simulink model "EV_compensated_system_via_detailed"  (R2016a)
settings: Solver=ode15s  StartTime=0.0  StopTime=tstop  MaxStep=1e-3  RelTol=1e-3
values from neighbouring files (symbols this model uses):
  Av = 2.16    [sim_parameters_via_motor_eff_data_improved.m]
  C = 500e-6    (= 0.0005)    [sim_parameters_via_motor_eff_data_improved.m]
  Cd = 0.26    [sim_parameters_via_motor_eff_data_improved.m]
  Cnom = 10    [sim_parameters_via_motor_eff_data_improved.m]
  Cr = 0.01    [sim_parameters_via_motor_eff_data_improved.m]
  etaC = 0.995    [sim_parameters_via_motor_eff_data_improved.m]
  Fv_max = Te_max*gratio/rw    (= 3970)    [sim_parameters_via_motor_eff_data_improved.m]
  Gci0 = Gciwc/abs(1+wzc/(i*wc))    [sim_parameters_via_motor_eff_data_improved.m]
  Gcm = 1000    [sim_parameters_via_motor_eff_data_improved.m]
  Gcv0 = Gcvwv/abs(1+wzo/(i*wv))    [sim_parameters_via_motor_eff_data_improved.m]
  gratio = 7.94    [sim_parameters_via_motor_eff_data_improved.m]
  H = 1/100    (= 0.01)    [sim_parameters_via_motor_eff_data_improved.m]
  Kp = Gciabs1/abs(1+wz1/(2*pi*10))    [sim_parameters_via_motor_eff_data_improved.m]
  L = 150e-6    (= 0.00015)    [sim_parameters_via_motor_eff_data_improved.m]
  L1 = 0.5e-3    (= 0.0005)    [sim_parameters_via_motor_eff_data_improved.m]
  lambda_m = 0.125    [sim_parameters_via_motor_eff_data_improved.m]
  Mp = 3    [sim_parameters_via_motor_eff_data_improved.m]
  Mv = 1250 + 55 + 15 + Ns*Mp*weight_cell    (= 1470)    [sim_parameters_via_motor_eff_data_improved.m]
  Ns = 100    [sim_parameters_via_motor_eff_data_improved.m]
  P = 8    [sim_parameters_via_motor_eff_data_improved.m]
  r = 0.04    [sim_parameters_via_motor_eff_data_improved.m]
  R1 = 5e-3    (= 0.005)    [sim_parameters_via_motor_eff_data_improved.m]
  rho_air = 1.204    [sim_parameters_via_motor_eff_data_improved.m]
  Rn = 5e-3    (= 0.005)    [sim_parameters_via_motor_eff_data_improved.m]
  Rp = 5e-3    (= 0.005)    [sim_parameters_via_motor_eff_data_improved.m]
  Rs = 1    [sim_parameters_via_motor_eff_data_improved.m]
  rw = 0.4    [sim_parameters_via_motor_eff_data_improved.m]
  SOC_0 = 0.75    [sim_parameters_via_motor_eff_data_improved.m]
  SOC_1 = 0.95    [sim_parameters_via_motor_eff_data_improved.m]
  tau1 = 240    [sim_parameters_via_motor_eff_data_improved.m]
  tauh = 40    [sim_parameters_via_motor_eff_data_improved.m]
  tstop = 750    [sim_parameters_via_motor_eff_data_improved.m]
  V_soc = [3.00205286349 3.0032462723 3.00443676789 3.00562435755 3.00680904852 3.00799084805 3.00916976335 3.01034580163 3.01151897006 3.01268927583 3.01385672607 3.0150213279 ... (9901 elements, 1x9901)]    [batt_V_SOC.mat]
  VM = 1    [sim_parameters_via_motor_eff_data_improved.m]
  Vm = 15e-3    (= 0.015)    [sim_parameters_via_motor_eff_data_improved.m]
  Vo = 600    [sim_parameters_via_motor_eff_data_improved.m]
  vref_1 = 6.7    [sim_parameters_via_motor_eff_data_improved.m]
  vref_2 = 8.9    [sim_parameters_via_motor_eff_data_improved.m]
  wz1 = wp    (= 80)    [sim_parameters_via_motor_eff_data_improved.m]
  wz2 = 2*pi*fz2    (= 0.00308184685714)    [sim_parameters_via_motor_eff_data_improved.m]
  wzc = 2*pi*fzc    (= 2513.27412287)    [sim_parameters_via_motor_eff_data_improved.m]
  wzo = 2*pi*fzo    (= 418.879020479)    [sim_parameters_via_motor_eff_data_improved.m]
libraries: simulink x5
settings Model: Creator=Gorkem  LastModifiedBy=Gorkem
settings DebuggingCC: MaxConsecutiveZCsMsg=none

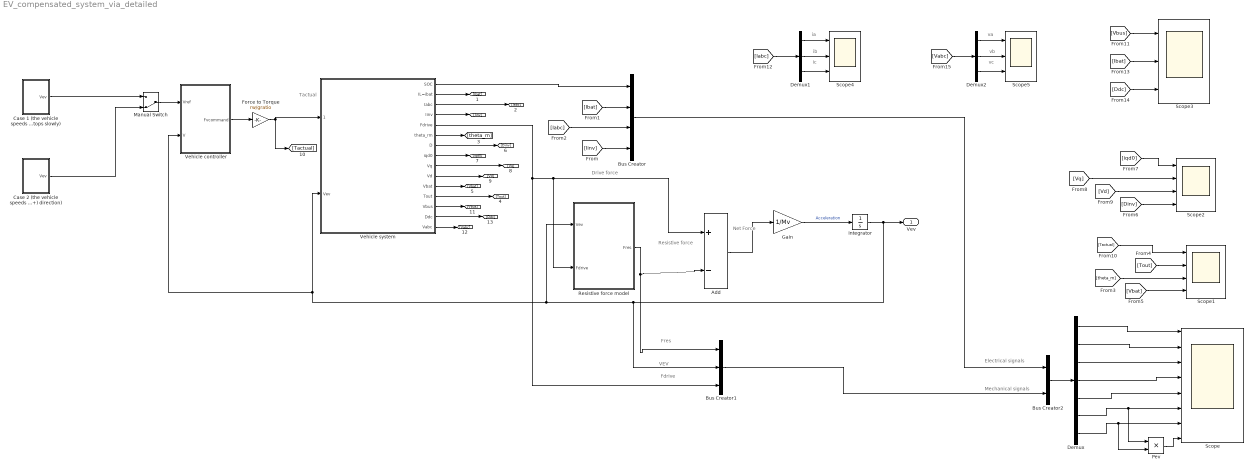
== system EV_compensated_system_via_detailed ==
  note: ic
  note: ib
  note: ia
  note: Fdrive
  note: VEV
  note: Fres
  note: Mechanical signals
  note: Electrical signals
  note: Resistive force
  note: Drive force
  note: Net
      | Force
  note: Tactual
  note: vc
  note: vb
  note: va
  Add : Sum  Inputs=+-
  Bus Creator : BusCreator  Inputs=4
  Bus Creator1 : BusCreator  Inputs=3
  Bus Creator2 : BusCreator  Inputs=2
  "Case 1 (the vehicle speeds up (+) direction  at first, then stops slowly)" : Subsystem
  "Case 2 (the vehicle speeds up in (-) direction at first, then stops slower and gets faster in (+) direction)" : Subsystem
  Demux : Demux  Outputs=7
  Demux1 : Demux  Outputs=3
  Demux2 : Demux  Outputs=3
  Force to Torque : Gain  Gain=rw/gratio
  Gain : Gain  Gain=1/Mv
  Integrator : Integrator
  Manual Switch : ManualSwitch  CurrentSetting=0
  Pev : Product
  Resistive force model : Subsystem
  Scope : Scope  NumInputPorts=8
  Scope1 : Scope  NumInputPorts=4
  Scope2 : Scope  NumInputPorts=4
  Scope3 : Scope  NumInputPorts=3
  Scope4 : Scope  NumInputPorts=3
  Scope5 : Scope  NumInputPorts=3
  Vehicle controller : Subsystem
  Vehicle system : Subsystem
  " Vev" : Outport
  wires:
  Add/1 -> Gain/1
  Gain/1 -> Integrator/1  "Acceleration"
  Vehicle system/5(Fdrive) -> Bus Creator1/3, Add/1, Resistive force model/2("Fdrive ")
  Resistive force model/1(Fres) -> Add/2, Bus Creator1/1
  Vehicle system/1(SOC) -> Bus Creator/1
  Bus Creator/1 -> Bus Creator2/1
  Bus Creator1/1 -> Bus Creator2/2
  Bus Creator2/1 -> Demux/1
  Demux/1 -> Scope/1
  Demux/2 -> Scope/2
  Demux/3 -> Scope/3
  Demux/4 -> Scope/4
  Demux/5 -> Scope/5
  Demux/6 -> Pev/1, Scope/6
  Demux/7 -> Pev/2, Scope/7
  Integrator/1 -> Bus Creator1/2, Resistive force model/1("Vev "), Vehicle system/2(Vev), Vehicle controller/2(V), " Vev"/1
  Vehicle controller/1(Fvcommand) -> Force to Torque/1
  Pev/1 -> Scope/8
  Force to Torque/1 -> Vehicle system/1(" "), [Tactual]
  Vehicle system/4(Iinv) -> [Iinv]
  [Iinv] -> Bus Creator/4
  Vehicle system/2(IL=ibat) -> [Ibat]
  [Ibat] -> Bus Creator/2
  Vehicle system/3(Iabc) -> [Iabc]
  Vehicle system/6(theta_rm) -> [theta_m]
  [theta_m] -> Scope1/3
  Vehicle system/12(Tout) -> [Tout]
  [Tout] -> Scope1/2
  Vehicle system/11(Vbat) -> [Vbat]
  [Vbat] -> Scope1/4
  Vehicle system/7(D) -> [Dinv]
  [Dinv] -> Scope2/4
  Vehicle system/8(iqd0) -> [iqd0]
  [iqd0] -> Scope2/1
  Vehicle system/9(Vq) -> [Vq]
  [Vq] -> Scope2/2
  Vehicle system/10(Vd) -> [Vd]
  [Vd] -> Scope2/3
  [Tactual] -> Scope1/1
  Vehicle system/13(Vbus) -> [Vbus]
  [Vbus] -> Scope3/1
  [Iabc] -> Bus Creator/3
  [Iabc] -> Demux1/1
  Demux1/1 -> Scope4/1
  Demux1/3 -> Scope4/3
  Demux1/2 -> Scope4/2
  [Ibat] -> Scope3/2
  Vehicle system/14(Ddc) -> [Ddc]
  [Ddc] -> Scope3/3
  Vehicle system/15(Vabc) -> [Vabc]
  [Vabc] -> Demux2/1
  Demux2/1 -> Scope5/1
  Demux2/3 -> Scope5/3
  Demux2/2 -> Scope5/2
  "Case 1 (the vehicle speeds up (+) direction  at first, then stops slowly)"/1("Vev ") -> Manual Switch/1
  "Case 2 (the vehicle speeds up in (-) direction at first, then stops slower and gets faster in (+) direction)"/1("Vev ") -> Manual Switch/2
  Manual Switch/1 -> Vehicle controller/1(Vref)

== system EV_compensated_system_via_detailed/Case 1 (the vehicle speeds up (+) direction  at first, then stops slowly) ==
  Add1 : Sum  Inputs=++++
  speed 1 : Step  Time=tstop/5  Before=vref_1  After=vref_2  SampleTime=0
  speed 2 : Step  Time=2*(tstop/5)  After=-vref_2+vref_1  SampleTime=0
  speed 5 : Step  Time=3*(tstop/5)  After=-vref_1/2  SampleTime=0
  speed 6 : Step  Time=4*(tstop/5)  After=-vref_1/2  SampleTime=0
  "Vev " : Outport
  wires:
  speed 2/1 -> Add1/2
  speed 6/1 -> Add1/4
  Add1/1 -> "Vev "/1
  speed 5/1 -> Add1/3
  speed 1/1 -> Add1/1

== system EV_compensated_system_via_detailed/Case 2 (the vehicle speeds up in (-) direction at first, then stops slower and gets faster in (+) direction) ==
  Add1 : Sum  Inputs=++++++
  speed 1 : Step  Time=tstop/7  Before=-vref_1/2  After=-vref_2/2  SampleTime=0
  speed 2 : Step  Time=2*(tstop/7)  After=vref_2/4  SampleTime=0
  speed 3 : Step  Time=5*(tstop/7)  After=vref_1/4  SampleTime=0
  speed 4 : Step  Time=6*(tstop/7)  After=(vref_2-vref_1)/2  SampleTime=0
  speed 5 : Step  Time=3*(tstop/7)  After=vref_2/4  SampleTime=0
  speed 6 : Step  Time=4*(tstop/7)  After=vref_1/4  SampleTime=0
  "Vev " : Outport
  wires:
  speed 2/1 -> Add1/2
  speed 6/1 -> Add1/4
  Add1/1 -> "Vev "/1
  speed 5/1 -> Add1/3
  speed 1/1 -> Add1/1
  speed 3/1 -> Add1/5
  speed 4/1 -> Add1/6

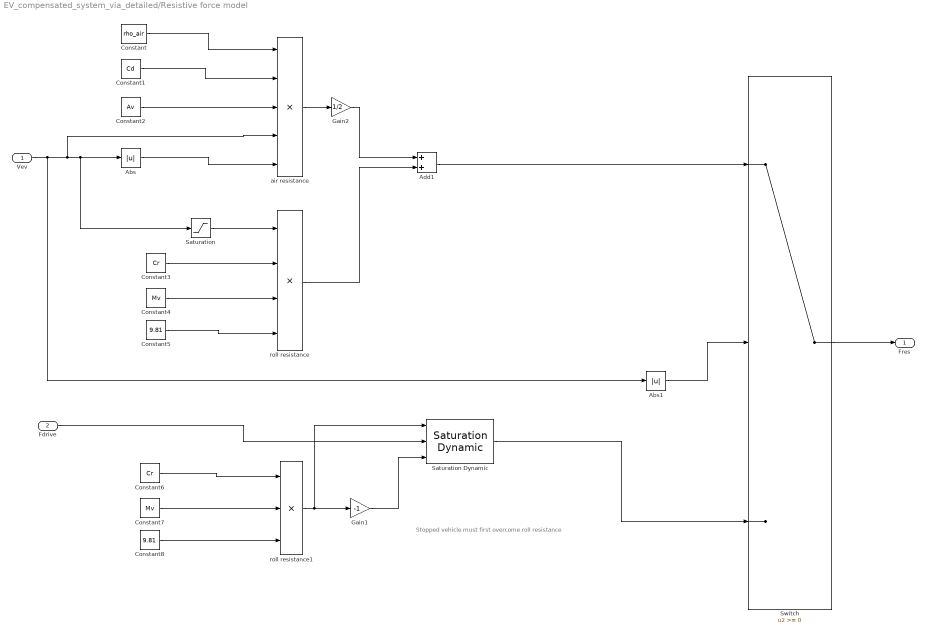
== system EV_compensated_system_via_detailed/Resistive force model ==
  note: Stopped vehicle must first overcome roll resistance
  "Vev " : Inport
  "Fdrive " : Inport  Port=2
  Abs : Abs  ZeroCross=off
  Abs1 : Abs
  Add1 : Sum
  Constant : Constant  Value=rho_air
  Constant1 : Constant  Value=Cd
  Constant2 : Constant  Value=Av
  Constant3 : Constant  Value=Cr
  Constant4 : Constant  Value=Mv
  Constant5 : Constant  Value=9.81
  Constant6 : Constant  Value=Cr
  Constant7 : Constant  Value=Mv
  Constant8 : Constant  Value=9.81
  Gain1 : Gain  Gain=-1
  Gain2 : Gain  Gain=1/2
  Saturation : Saturate  UpperLimit=1  LowerLimit=-1
  Saturation Dynamic : simulink/Discontinuities/Saturation Dynamic  OutMin=[]  OutMax=[]  OutDataTypeStr=Inherit: Same as second input  OutDataType=fixdt(1, 16)  OutScaling=2^-10  DoSatur=off
  Switch : Switch  ZeroCross=off
  "air resistance " : Product  Inputs=5
  roll resistance : Product  Inputs=4
  roll resistance1 : Product  Inputs=3
  Fres : Outport
  wires:
  Saturation Dynamic/1 -> Switch/3
  Constant2/1 -> "air resistance "/3
  Constant8/1 -> roll resistance1/3
  Gain2/1 -> Add1/1
  Constant4/1 -> roll resistance/3
  Constant1/1 -> "air resistance "/2
  Constant6/1 -> roll resistance1/1
  Constant3/1 -> roll resistance/2
  "Vev "/1 -> Abs1/1, "air resistance "/4, Saturation/1, Abs/1
  Constant/1 -> "air resistance "/1
  Constant5/1 -> roll resistance/4
  Saturation/1 -> roll resistance/1
  "air resistance "/1 -> Gain2/1
  roll resistance/1 -> Add1/2
  Constant7/1 -> roll resistance1/2
  Gain1/1 -> Saturation Dynamic/3
  Add1/1 -> Switch/1
  Abs1/1 -> Switch/2
  Switch/1 -> Fres/1
  roll resistance1/1 -> Saturation Dynamic/1, Gain1/1
  Abs/1 -> "air resistance "/5
  "Fdrive "/1 -> Saturation Dynamic/2

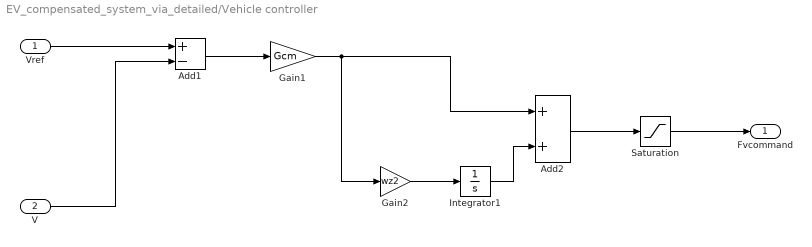
== system EV_compensated_system_via_detailed/Vehicle controller ==
  Vref : Inport
  V : Inport  Port=2
  Add1 : Sum  Inputs=+-
  Add2 : Sum
  Gain1 : Gain  Gain=Gcm
  Gain2 : Gain  Gain=wz2
  Integrator1 : Integrator
  Saturation : Saturate  UpperLimit=Fv_max  LowerLimit=-Fv_max
  Fvcommand : Outport
  wires:
  Gain1/1 -> Add2/1, Gain2/1
  Gain2/1 -> Integrator1/1
  Integrator1/1 -> Add2/2
  V/1 -> Add1/2
  Add1/1 -> Gain1/1
  Add2/1 -> Saturation/1
  Vref/1 -> Add1/1
  Saturation/1 -> Fvcommand/1

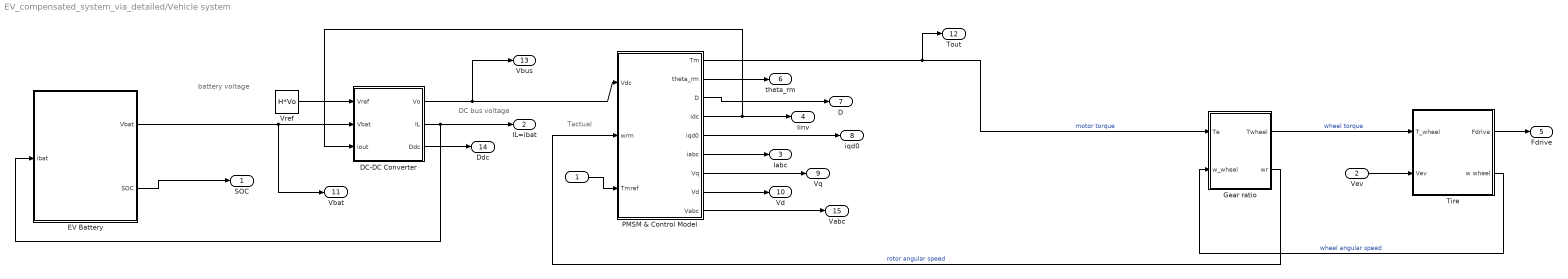
== system EV_compensated_system_via_detailed/Vehicle system ==
  note: DC bus voltage
  note: Tactual
  note: battery voltage
  " " : Inport
  Vev : Inport  Port=2
  DC-DC Converter : Subsystem
  EV Battery : Subsystem
  Gear ratio : Subsystem
  PMSM & Control Model : Subsystem
  Tire : Subsystem
  Vref : Constant  Value=H*Vo
  SOC : Outport
  IL=ibat : Outport  Port=2
  Iabc : Outport  Port=3
  Iinv : Outport  Port=4
  Fdrive : Outport  Port=5
  theta_rm : Outport  Port=6
  D : Outport  Port=7
  iqd0 : Outport  Port=8
  Vq : Outport  Port=9
  Vd : Outport  Port=10
  Vbat : Outport  Port=11
  Tout : Outport  Port=12
  Vbus : Outport  Port=13
  Ddc : Outport  Port=14
  Vabc : Outport  Port=15
  wires:
  Gear ratio/1(Twheel) -> Tire/1(T_wheel)  "wheel torque"
  " "/1 -> PMSM & Control Model/3(Tmref)
  EV Battery/1(Vbat) -> Vbat/1, DC-DC Converter/2(Vbat)
  PMSM & Control Model/1(Tm) -> Tout/1, Gear ratio/1(Te)  "motor torque"
  DC-DC Converter/1(Vo) -> Vbus/1, PMSM & Control Model/1(Vdc)
  EV Battery/2(SOC) -> SOC/1
  Vev/1 -> Tire/2(Vev)
  Tire/1(Fdrive) -> Fdrive/1
  PMSM & Control Model/6(iabc) -> Iabc/1
  Vref/1 -> DC-DC Converter/1(Vref)
  PMSM & Control Model/4(idc) -> Iinv/1, DC-DC Converter/3(iout)
  PMSM & Control Model/2(theta_rm) -> theta_rm/1
  PMSM & Control Model/3(D) -> D/1
  PMSM & Control Model/5(iqd0) -> iqd0/1
  PMSM & Control Model/7(Vq) -> Vq/1
  PMSM & Control Model/8(Vd) -> Vd/1
  Gear ratio/2(wr) -> PMSM & Control Model/2(wrm)  "rotor angular speed"
  Tire/2(w wheel) -> Gear ratio/2(w_wheel)  "wheel angular speed"
  DC-DC Converter/3(Ddc) -> Ddc/1
  DC-DC Converter/2(IL) -> EV Battery/1(ibat), IL=ibat/1
  PMSM & Control Model/9(Vabc) -> Vabc/1

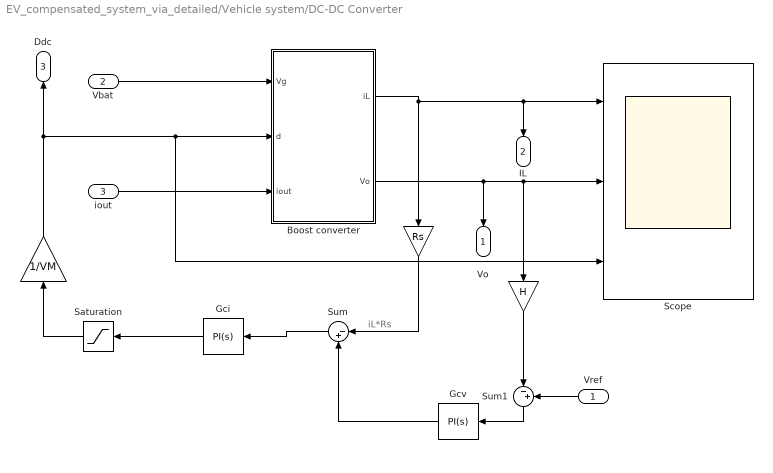
== system EV_compensated_system_via_detailed/Vehicle system/DC-DC Converter ==
  note: iL*Rs
  Vref : Inport
  Vbat : Inport  Port=2
  iout : Inport  Port=3
  "  " : Gain  Gain=Rs
  "     " : Gain  Gain=1/VM
  "           " : Gain  Gain=H
  Boost converter : Subsystem
  Gci : simulink/Continuous/PID Controller  Controller=PI  TimeDomain=Continuous-time  SampleTime=-1  IntegratorMethod=Forward Euler  FilterMethod=Forward Euler  Form=Parallel  UseFilter=on  ControllerParametersSource=internal  P=Gci0  I=Gci0*wzc  D=0  N=100  InitialConditionSource=internal  InitialConditionForIntegrator=0  InitialConditionForFilter=0  ExternalReset=none  LimitOutput=off  UpperSaturationLimit=inf  LowerSaturationLimit=-inf  LinearizeAsGain=on  AntiWindupMode=none  Kb=1  TrackingMode=off  Kt=1  PParamMin=[]  PParamMax=[]  IParamMin=[]  IParamMax=[]  DParamMin=[]  DParamMax=[]  NParamMin=[]  NParamMax=[]  KbParamMin=[]  KbParamMax=[]  KtParamMin=[]  KtParamMax=[]  POutMin=[]  POutMax=[]  IOutMin=[]  IOutMax=[]  DOutMin=[]  DOutMax=[]  NOutMin=[]  NOutMax=[]  KbOutMin=[]  KbOutMax=[]  KtOutMin=[]  KtOutMax=[]  IntegratorOutMin=[]  IntegratorOutMax=[]  FilterOutMin=[]  FilterOutMax=[]  SumOutMin=[]  SumOutMax=[]  SumI1OutMin=[]  SumI1OutMax=[]  SumI2OutMin=[]  SumI2OutMax=[]  SumI3OutMin=[]  SumI3OutMax=[]  SumDOutMin=[]  SumDOutMax=[]  SaturationOutMin=[]  SaturationOutMax=[]  IntegratorContinuousStateAttributes=''  IntegratorStateMustResolveToSignalObject=off  IntegratorRTWStateStorageClass=Auto  FilterContinuousStateAttributes=''  FilterStateMustResolveToSignalObject=off  FilterRTWStateStorageClass=Auto  DifferentiatorICPrevScaledInput=0  DifferentiatorOutMin=[]  DifferentiatorOutMax=[]
  Gcv : simulink/Continuous/PID Controller  Controller=PI  TimeDomain=Continuous-time  SampleTime=-1  IntegratorMethod=Forward Euler  FilterMethod=Forward Euler  Form=Parallel  UseFilter=on  ControllerParametersSource=internal  P=Gcv0  I=Gcv0*wzo  D=0  N=100  InitialConditionSource=internal  InitialConditionForIntegrator=0  InitialConditionForFilter=0  ExternalReset=none  LimitOutput=off  UpperSaturationLimit=inf  LowerSaturationLimit=-inf  LinearizeAsGain=on  AntiWindupMode=none  Kb=1  TrackingMode=off  Kt=1  PParamMin=[]  PParamMax=[]  IParamMin=[]  IParamMax=[]  DParamMin=[]  DParamMax=[]  NParamMin=[]  NParamMax=[]  KbParamMin=[]  KbParamMax=[]  KtParamMin=[]  KtParamMax=[]  POutMin=[]  POutMax=[]  IOutMin=[]  IOutMax=[]  DOutMin=[]  DOutMax=[]  NOutMin=[]  NOutMax=[]  KbOutMin=[]  KbOutMax=[]  KtOutMin=[]  KtOutMax=[]  IntegratorOutMin=[]  IntegratorOutMax=[]  FilterOutMin=[]  FilterOutMax=[]  SumOutMin=[]  SumOutMax=[]  SumI1OutMin=[]  SumI1OutMax=[]  SumI2OutMin=[]  SumI2OutMax=[]  SumI3OutMin=[]  SumI3OutMax=[]  SumDOutMin=[]  SumDOutMax=[]  SaturationOutMin=[]  SaturationOutMax=[]  IntegratorContinuousStateAttributes=''  IntegratorStateMustResolveToSignalObject=off  IntegratorRTWStateStorageClass=Auto  FilterContinuousStateAttributes=''  FilterStateMustResolveToSignalObject=off  FilterRTWStateStorageClass=Auto  DifferentiatorICPrevScaledInput=0  DifferentiatorOutMin=[]  DifferentiatorOutMax=[]
  Saturation : Saturate  UpperLimit=1  LowerLimit=0
  Scope : Scope  NumInputPorts=3
  Sum : Sum  Inputs=|-+
  Sum1 : Sum  Inputs=|-+
  Vo : Outport
  IL : Outport  Port=2
  Ddc : Outport  Port=3
  wires:
  Vbat/1 -> Boost converter/1(Vg)
  Gci/1 -> Saturation/1
  Boost converter/2(Vo) -> Vo/1, "           "/1, Scope/2
  Gcv/1 -> Sum/2
  Sum/1 -> Gci/1
  iout/1 -> Boost converter/3(iout)
  Saturation/1 -> "     "/1
  "  "/1 -> Sum/1
  "           "/1 -> Sum1/1
  Sum1/1 -> Gcv/1
  "     "/1 -> Ddc/1, Scope/3, Boost converter/2(d)
  Vref/1 -> Sum1/2
  Boost converter/1(iL) -> IL/1, Scope/1, "  "/1

== system EV_compensated_system_via_detailed/Vehicle system/EV Battery ==
  note: Ebat
  note: Pbat
  ibat : Inport
  Integrator : Integrator
  Li-ion Battery : Subsystem
  Product : Product
  Scope : Scope  NumInputPorts=4
  "ibat>0, discharging, Pbat<0 ibat<0, charging, Pbat>0" : Gain  Gain=-1
  Vbat : Outport
  SOC : Outport  Port=2
  wires:
  Integrator/1 -> Scope/4
  Li-ion Battery/2(SOC) -> SOC/1, Scope/2
  Product/1 -> Integrator/1
  "ibat>0, discharging, Pbat<0 ibat<0, charging, Pbat>0"/1 -> Product/2
  Li-ion Battery/1(Vbat) -> Product/1, Vbat/1, Scope/1
  ibat/1 -> Scope/3, "ibat>0, discharging, Pbat<0 ibat<0, charging, Pbat>0"/1, Li-ion Battery/1(ibat)

== system EV_compensated_system_via_detailed/Vehicle system/Gear ratio ==
  Te : Inport
  w_wheel : Inport  Port=2
  Constant : Constant  Value=gratio
  Product : Product
  Product1 : Product
  Twheel : Outport
  wr : Outport  Port=2
  wires:
  Product/1 -> Twheel/1
  Constant/1 -> Product1/1, Product/2
  Te/1 -> Product/1
  Product1/1 -> wr/1
  w_wheel/1 -> Product1/2

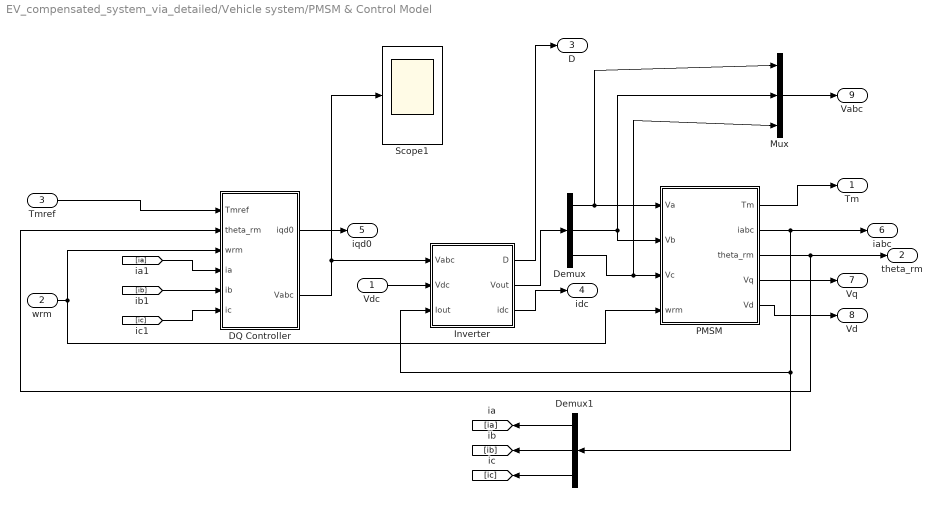
== system EV_compensated_system_via_detailed/Vehicle system/PMSM & Control Model ==
  Vdc : Inport
  wrm : Inport  Port=2
  Tmref : Inport  Port=3
  DQ Controller : Subsystem
  Demux : Demux  Outputs=3
  Demux1 : Demux  Outputs=3
  Inverter : Subsystem
  Mux : Mux  Inputs=3
  PMSM : Subsystem
  Scope1 : Scope
  Tm : Outport
  theta_rm : Outport  Port=2
  D : Outport  Port=3
  idc : Outport  Port=4
  iqd0 : Outport  Port=5
  iabc : Outport  Port=6
  Vq : Outport  Port=7
  Vd : Outport  Port=8
  Vabc : Outport  Port=9
  wires:
  DQ Controller/2(Vabc) -> Scope1/1, Inverter/1(Vabc)
  Inverter/1(D) -> D/1
  Demux/3 -> Mux/3, PMSM/3(Vc)
  PMSM/3(theta_rm) -> DQ Controller/2(theta_rm), theta_rm/1
  Inverter/3(idc) -> idc/1
  Tmref/1 -> DQ Controller/1(Tmref)
  wrm/1 -> PMSM/4(wrm), DQ Controller/3(wrm)
  DQ Controller/1(iqd0) -> iqd0/1
  Demux/2 -> Mux/2, PMSM/2(Vb)
  Inverter/2(Vout) -> Demux/1
  PMSM/1(Tm) -> Tm/1
  Demux/1 -> Mux/1, PMSM/1(Va)
  PMSM/4(Vq) -> Vq/1
  PMSM/5(Vd) -> Vd/1
  PMSM/2("iabc ") -> Demux1/1, Inverter/3("Iout "), iabc/1
  Demux1/1 -> [ia]
  Demux1/2 -> [ib]
  Demux1/3 -> [ic]
  [ia] -> DQ Controller/4(ia)
  [ib] -> DQ Controller/5(ib)
  [ic] -> DQ Controller/6(ic)
  Vdc/1 -> Inverter/2(Vdc)
  Mux/1 -> Vabc/1

== system EV_compensated_system_via_detailed/Vehicle system/Tire ==
  T_wheel : Inport
  Vev : Inport  Port=2
  Gain : Gain  Gain=1/rw
  Gain1 : Gain  Gain=1/rw
  Fdrive : Outport
  w wheel : Outport  Port=2
  wires:
  T_wheel/1 -> Gain/1
  Gain/1 -> Fdrive/1
  Vev/1 -> Gain1/1
  Gain1/1 -> w wheel/1

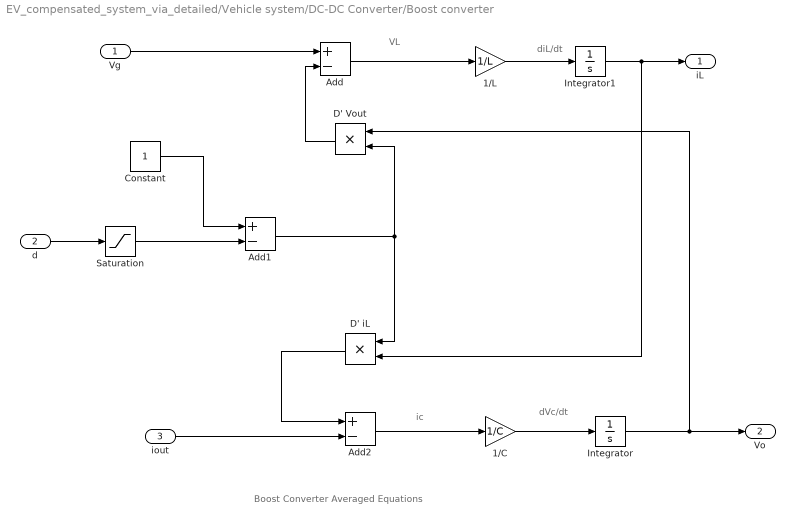
== system EV_compensated_system_via_detailed/Vehicle system/DC-DC Converter/Boost converter ==
  note: Boost Converter Averaged Equations
  note: dVc/dt
  note: ic
  note: diL/dt
  note: VL
  Vg : Inport
  d : Inport  Port=2
  iout : Inport  Port=3
  1/C : Gain  Gain=1/C
  1/L : Gain  Gain=1/L
  Add : Sum  Inputs=+-
  Add1 : Sum  Inputs=+-
  Add2 : Sum  Inputs=+-
  Constant : Constant
  D' Vout : Product
  D' iL : Product
  Integrator : Integrator
  Integrator1 : Integrator
  Saturation : Saturate  UpperLimit=1  LowerLimit=0
  iL : Outport
  Vo : Outport  Port=2
  wires:
  d/1 -> Saturation/1
  Constant/1 -> Add1/1
  Integrator/1 -> D' Vout/1, Vo/1
  Add1/1 -> D' Vout/2, D' iL/1
  D' Vout/1 -> Add/2
  Vg/1 -> Add/1
  Add/1 -> 1/L/1
  1/L/1 -> Integrator1/1
  Integrator1/1 -> D' iL/2, iL/1
  D' iL/1 -> Add2/1
  iout/1 -> Add2/2
  Add2/1 -> 1/C/1
  1/C/1 -> Integrator/1
  Saturation/1 -> Add1/2

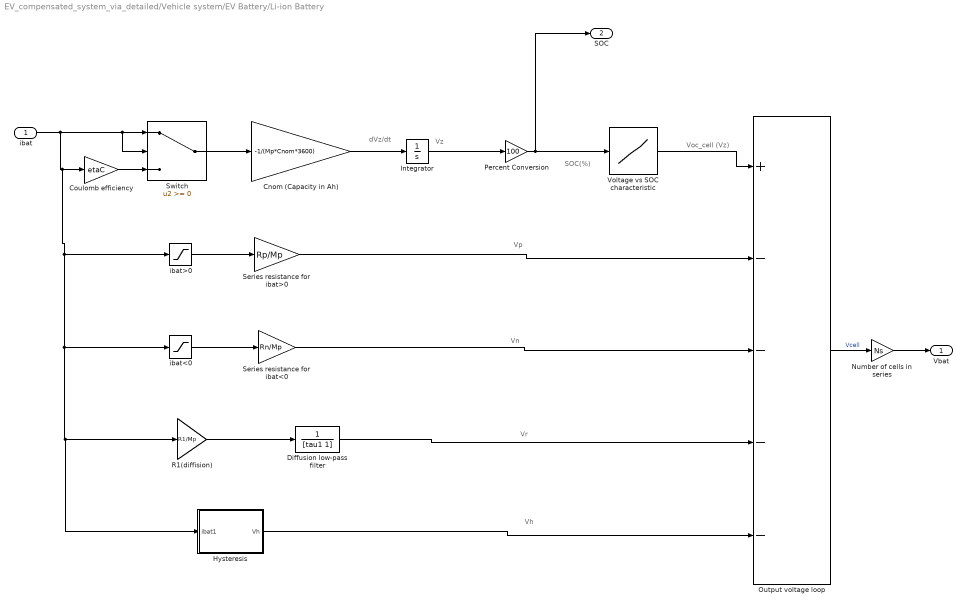
== system EV_compensated_system_via_detailed/Vehicle system/EV Battery/Li-ion Battery ==
  note: Voc_cell (Vz)
  note: SOC(%)
  note: Vz
  note: Vh
  note: Vr
  note: Vn
  note: Vp
  note: dVz/dt
  ibat : Inport
  Cnom (Capacity in Ah) : Gain  Gain=-1/(Mp*Cnom*3600)
  Coulomb efficiency : Gain  Gain=etaC
  Diffusion low-pass filter : TransferFcn  Denominator=[tau1 1]
  Hysteresis : Subsystem
  Integrator : Integrator  InitialCondition=SOC_0  LimitOutput=on  UpperSaturationLimit=SOC_1  LowerSaturationLimit=SOC_0/2.5
  Number of cells in series : Gain  Gain=Ns
  Output voltage loop : Sum  Inputs=+----
  "Percent Conversion " : Gain  Gain=100
  R1(diffision) : Gain  Gain=R1/Mp
  Series resistance for ibat<0 : Gain  Gain=Rn/Mp
  Series resistance for ibat>0 : Gain  Gain=Rp/Mp
  Switch : Switch
  Voltage vs SOC characteristic : Lookup_n-D  NumberOfTableDimensions=1  BreakpointsForDimension1=[0:9900]/100  Table=V_soc  InternalRulePriority=Speed  RndMeth=Simplest  InputSameDT=on
  ibat<0 : Saturate  UpperLimit=0  LowerLimit=-inf
  ibat>0 : Saturate  UpperLimit=inf  LowerLimit=0
  Vbat : Outport
  SOC : Outport  Port=2
  wires:
  R1(diffision)/1 -> Diffusion low-pass filter/1
  Diffusion low-pass filter/1 -> Output voltage loop/4
  Series resistance for ibat>0/1 -> Output voltage loop/2
  Series resistance for ibat<0/1 -> Output voltage loop/3
  Hysteresis/1(Vh) -> Output voltage loop/5
  ibat/1 -> Hysteresis/1(ibat1), R1(diffision)/1, ibat<0/1, ibat>0/1, Coulomb efficiency/1, Switch/2, Switch/1
  Number of cells in series/1 -> Vbat/1
  Output voltage loop/1 -> Number of cells in series/1  "Vcell"
  Voltage vs SOC characteristic/1 -> Output voltage loop/1
  ibat>0/1 -> Series resistance for ibat>0/1
  Coulomb efficiency/1 -> Switch/3
  Switch/1 -> Cnom (Capacity in Ah)/1
  Cnom (Capacity in Ah)/1 -> Integrator/1
  ibat<0/1 -> Series resistance for ibat<0/1
  "Percent Conversion "/1 -> SOC/1, Voltage vs SOC characteristic/1
  Integrator/1 -> "Percent Conversion "/1

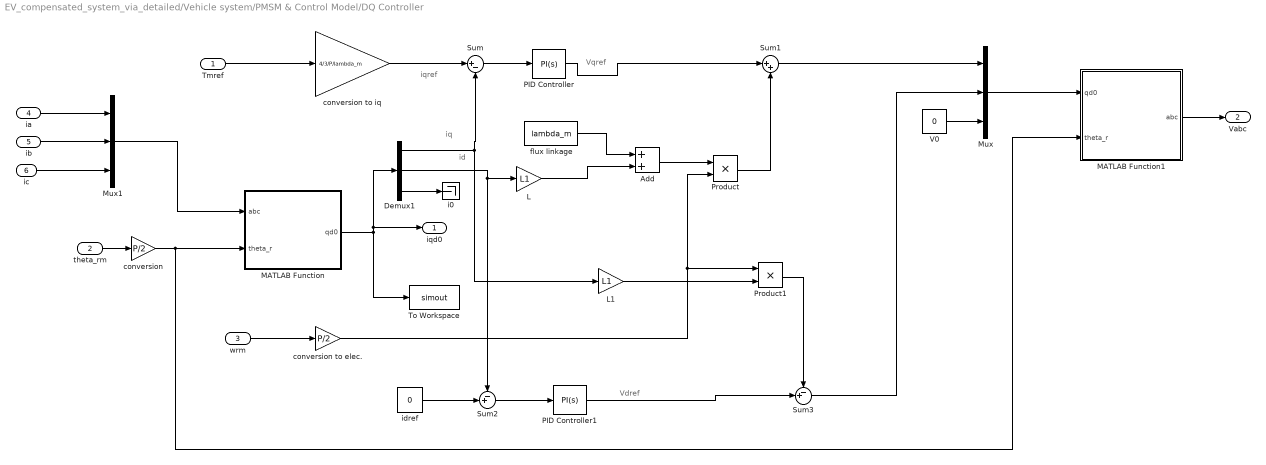
== system EV_compensated_system_via_detailed/Vehicle system/PMSM & Control Model/DQ Controller ==
  note: iqref
  note: Vdref
  note: id
  note: Vqref
  note: iq
  Tmref : Inport
  theta_rm : Inport  Port=2
  wrm : Inport  Port=3
  ia : Inport  Port=4
  ib : Inport  Port=5
  ic : Inport  Port=6
  Add : Sum
  Demux1 : Demux  Outputs=[1 1 1]
  L : Gain  Gain=L1
  L1 : Gain  Gain=L1
  MATLAB Function : MATLAB Function  TreatAsAtomicUnit=on
  MATLAB Function1 : MATLAB Function  TreatAsAtomicUnit=on
  Mux : Mux  Inputs=[1 1 1]
  Mux1 : Mux  Inputs=[1 1 1]
  PID Controller : simulink/Continuous/PID Controller  Controller=PI  TimeDomain=Continuous-time  SampleTime=-1  IntegratorMethod=Forward Euler  FilterMethod=Forward Euler  Form=Parallel  UseFilter=on  ControllerParametersSource=internal  P=Kp  I=Kp*wz1  D=0  N=100  InitialConditionSource=internal  InitialConditionForIntegrator=0  InitialConditionForFilter=0  ExternalReset=none  LimitOutput=off  UpperSaturationLimit=inf  LowerSaturationLimit=-inf  LinearizeAsGain=on  AntiWindupMode=none  Kb=1  TrackingMode=off  Kt=1  PParamMin=[]  PParamMax=[]  IParamMin=[]  IParamMax=[]  DParamMin=[]  DParamMax=[]  NParamMin=[]  NParamMax=[]  KbParamMin=[]  KbParamMax=[]  KtParamMin=[]  KtParamMax=[]  POutMin=[]  POutMax=[]  IOutMin=[]  IOutMax=[]  DOutMin=[]  DOutMax=[]  NOutMin=[]  NOutMax=[]  KbOutMin=[]  KbOutMax=[]  KtOutMin=[]  KtOutMax=[]  IntegratorOutMin=[]  IntegratorOutMax=[]  FilterOutMin=[]  FilterOutMax=[]  SumOutMin=[]  SumOutMax=[]  SumI1OutMin=[]  SumI1OutMax=[]  SumI2OutMin=[]  SumI2OutMax=[]  SumI3OutMin=[]  SumI3OutMax=[]  SumDOutMin=[]  SumDOutMax=[]  SaturationOutMin=[]  SaturationOutMax=[]  IntegratorContinuousStateAttributes=''  IntegratorStateMustResolveToSignalObject=off  IntegratorRTWStateStorageClass=Auto  FilterContinuousStateAttributes=''  FilterStateMustResolveToSignalObject=off  FilterRTWStateStorageClass=Auto  DifferentiatorICPrevScaledInput=0  DifferentiatorOutMin=[]  DifferentiatorOutMax=[]
  PID Controller1 : simulink/Continuous/PID Controller  Controller=PI  TimeDomain=Continuous-time  SampleTime=-1  IntegratorMethod=Forward Euler  FilterMethod=Forward Euler  Form=Parallel  UseFilter=on  ControllerParametersSource=internal  P=Kp  I=Kp*wz1  D=0  N=100  InitialConditionSource=internal  InitialConditionForIntegrator=0  InitialConditionForFilter=0  ExternalReset=none  LimitOutput=off  UpperSaturationLimit=inf  LowerSaturationLimit=-inf  LinearizeAsGain=on  AntiWindupMode=none  Kb=1  TrackingMode=off  Kt=1  PParamMin=[]  PParamMax=[]  IParamMin=[]  IParamMax=[]  DParamMin=[]  DParamMax=[]  NParamMin=[]  NParamMax=[]  KbParamMin=[]  KbParamMax=[]  KtParamMin=[]  KtParamMax=[]  POutMin=[]  POutMax=[]  IOutMin=[]  IOutMax=[]  DOutMin=[]  DOutMax=[]  NOutMin=[]  NOutMax=[]  KbOutMin=[]  KbOutMax=[]  KtOutMin=[]  KtOutMax=[]  IntegratorOutMin=[]  IntegratorOutMax=[]  FilterOutMin=[]  FilterOutMax=[]  SumOutMin=[]  SumOutMax=[]  SumI1OutMin=[]  SumI1OutMax=[]  SumI2OutMin=[]  SumI2OutMax=[]  SumI3OutMin=[]  SumI3OutMax=[]  SumDOutMin=[]  SumDOutMax=[]  SaturationOutMin=[]  SaturationOutMax=[]  IntegratorContinuousStateAttributes=''  IntegratorStateMustResolveToSignalObject=off  IntegratorRTWStateStorageClass=Auto  FilterContinuousStateAttributes=''  FilterStateMustResolveToSignalObject=off  FilterRTWStateStorageClass=Auto  DifferentiatorICPrevScaledInput=0  DifferentiatorOutMin=[]  DifferentiatorOutMax=[]
  Product : Product
  Product1 : Product
  Sum : Sum  Inputs=|+-
  Sum1 : Sum  Inputs=|++
  Sum2 : Sum  Inputs=-+|
  Sum3 : Sum  Inputs=-+|
  To Workspace : ToWorkspace  VariableName=simout  SaveFormat=Structure  SampleTime=-1
  V0 : Constant  Value=0
  "conversion " : Gain  Gain=P/2
  conversion to elec. : Gain  Gain=P/2
  conversion to iq : Gain  Gain=4/3/P/lambda_m
  flux linkage : Constant  Value=lambda_m
  i0 : Terminator
  idref : Constant  Value=0
  iqd0 : Outport
  Vabc : Outport  Port=2
  wires:
  wrm/1 -> conversion to elec./1
  theta_rm/1 -> "conversion "/1
  Tmref/1 -> conversion to iq/1
  MATLAB Function/1(qd0) -> Demux1/1, iqd0/1, To Workspace/1
  conversion to iq/1 -> Sum/1
  Demux1/1 -> Sum/2, L1/1
  Sum/1 -> PID Controller/1
  PID Controller/1 -> Sum1/1
  Demux1/2 -> L/1, Sum2/1
  L/1 -> Add/2
  flux linkage/1 -> Add/1
  Add/1 -> Product/1
  conversion to elec./1 -> Product/2, Product1/1
  Product/1 -> Sum1/2
  idref/1 -> Sum2/2
  Sum2/1 -> PID Controller1/1
  L1/1 -> Product1/2
  PID Controller1/1 -> Sum3/2
  Product1/1 -> Sum3/1
  Sum1/1 -> Mux/1
  V0/1 -> Mux/3
  "conversion "/1 -> MATLAB Function1/2(theta_r), MATLAB Function/2(theta_r)
  Demux1/3 -> i0/1
  Mux1/1 -> MATLAB Function/1(abc)
  Sum3/1 -> Mux/2
  Mux/1 -> MATLAB Function1/1(qd0)
  MATLAB Function1/1(abc) -> Vabc/1
  ia/1 -> Mux1/1
  ib/1 -> Mux1/2
  ic/1 -> Mux1/3

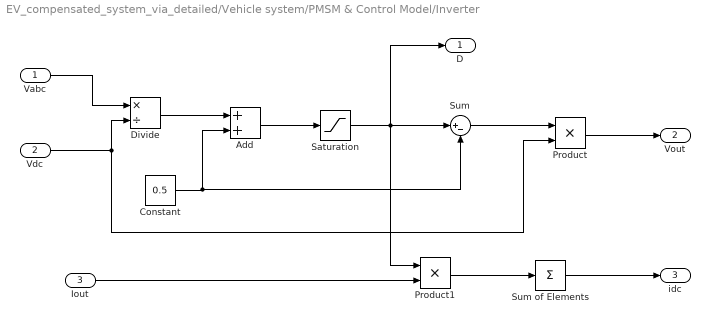
== system EV_compensated_system_via_detailed/Vehicle system/PMSM & Control Model/Inverter ==
  Vabc : Inport
  Vdc : Inport  Port=2
  "Iout " : Inport  Port=3
  Add : Sum
  Constant : Constant  Value=0.5
  Divide : Product  Inputs=*/
  Product : Product
  Product1 : Product
  Saturation : Saturate  UpperLimit=1  LowerLimit=0
  Sum : Sum  Inputs=|+-
  Sum of Elements : Sum  Inputs=+
  D : Outport
  Vout : Outport  Port=2
  idc : Outport  Port=3
  wires:
  Constant/1 -> Sum/2, Add/2
  Vabc/1 -> Divide/1
  Divide/1 -> Add/1
  Product/1 -> Vout/1
  Sum/1 -> Product/1
  "Iout "/1 -> Product1/2
  Product1/1 -> Sum of Elements/1
  Sum of Elements/1 -> idc/1
  Vdc/1 -> Divide/2, Product/2
  Saturation/1 -> D/1, Product1/1, Sum/1
  Add/1 -> Saturation/1

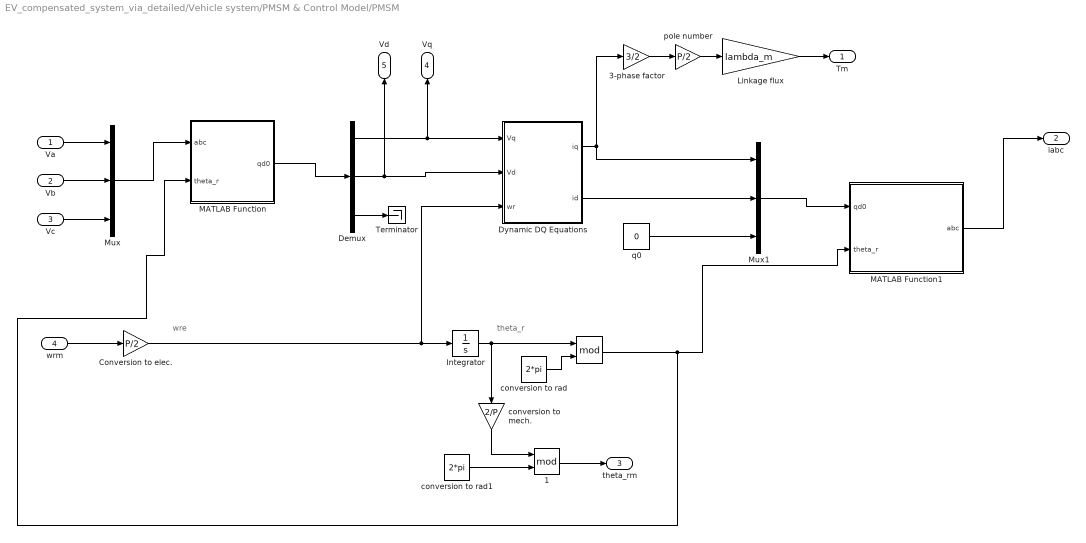
== system EV_compensated_system_via_detailed/Vehicle system/PMSM & Control Model/PMSM ==
  note: theta_r
  note: wre
  Va : Inport
  Vb : Inport  Port=2
  Vc : Inport  Port=3
  wrm : Inport  Port=4
  "  " : Math  Operator=mod  SaturateOnIntegerOverflow=on
  "  1" : Math  Operator=mod  SaturateOnIntegerOverflow=on
  3-phase factor : Gain  Gain=3/2
  Conversion to elec. : Gain  Gain=P/2
  Demux : Demux  Outputs=3
  Dynamic DQ Equations : Subsystem
  Integrator : Integrator
  Linkage flux : Gain  Gain=lambda_m
  MATLAB Function : MATLAB Function  TreatAsAtomicUnit=on
  MATLAB Function1 : MATLAB Function  TreatAsAtomicUnit=on
  Mux : Mux  Inputs=3
  Mux1 : Mux  Inputs=3
  Terminator : Terminator
  conversion to mech. : Gain  Gain=2/P
  conversion to rad : Constant  Value=2*pi
  conversion to rad1 : Constant  Value=2*pi
  pole number : Gain  Gain=P/2
  q0 : Constant  Value=0
  Tm : Outport
  "iabc " : Outport  Port=2
  theta_rm : Outport  Port=3
  Vq : Outport  Port=4
  Vd : Outport  Port=5
  wires:
  "  1"/1 -> theta_rm/1
  "  "/1 -> MATLAB Function/2(theta_r), MATLAB Function1/2(theta_r)
  conversion to mech./1 -> "  1"/1
  conversion to rad1/1 -> "  1"/2
  Integrator/1 -> "  "/1, conversion to mech./1
  MATLAB Function1/1(abc) -> "iabc "/1
  Vc/1 -> Mux/3
  Demux/1 -> Vq/1, Dynamic DQ Equations/1(Vq)
  Va/1 -> Mux/1
  q0/1 -> Mux1/3
  pole number/1 -> Linkage flux/1
  Dynamic DQ Equations/2(id) -> Mux1/2
  conversion to rad/1 -> "  "/2
  Demux/3 -> Terminator/1
  Vb/1 -> Mux/2
  Demux/2 -> Vd/1, Dynamic DQ Equations/2(Vd)
  Dynamic DQ Equations/1(iq) -> Mux1/1, 3-phase factor/1
  Conversion to elec./1 -> Dynamic DQ Equations/3(wr), Integrator/1
  wrm/1 -> Conversion to elec./1
  3-phase factor/1 -> pole number/1
  Linkage flux/1 -> Tm/1
  MATLAB Function/1(qd0) -> Demux/1
  Mux/1 -> MATLAB Function/1(abc)
  Mux1/1 -> MATLAB Function1/1(qd0)

== system EV_compensated_system_via_detailed/Vehicle system/EV Battery/Li-ion Battery/Hysteresis ==
  ibat1 : Inport
  Hysteresis state : TransferFcn  Denominator=[tauh 1]
  Relay : Relay  OnSwitchValue=0.01  OffSwitchValue=-0.01  OnOutputValue=Vm  OffOutputValue=-Vm
  Vh : Outport
  wires:
  Relay/1 -> Hysteresis state/1
  ibat1/1 -> Relay/1
  Hysteresis state/1 -> Vh/1

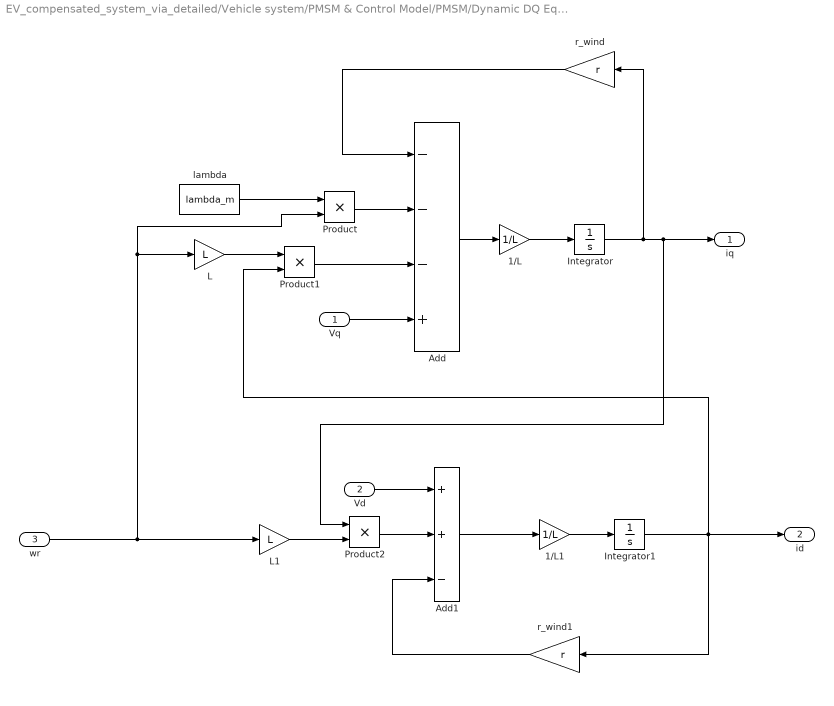
== system EV_compensated_system_via_detailed/Vehicle system/PMSM & Control Model/PMSM/Dynamic DQ Equations ==
  Vq : Inport
  Vd : Inport  Port=2
  wr : Inport  Port=3
  1/L : Gain  Gain=1/L
  1/L1 : Gain  Gain=1/L
  Add : Sum  Inputs=---+
  Add1 : Sum  Inputs=++-
  Integrator : Integrator
  Integrator1 : Integrator
  L : Gain  Gain=L
  L1 : Gain  Gain=L
  Product : Product
  Product1 : Product
  Product2 : Product
  lambda : Constant  Value=lambda_m
  r_wind : Gain  Gain=r
  r_wind1 : Gain  Gain=r
  iq : Outport
  id : Outport  Port=2
  wires:
  1/L/1 -> Integrator/1
  Vq/1 -> Add/4
  r_wind/1 -> Add/1
  Integrator1/1 -> id/1, r_wind1/1, Product1/2
  Vd/1 -> Add1/1
  r_wind1/1 -> Add1/3
  Product1/1 -> Add/3
  Add/1 -> 1/L/1
  Product2/1 -> Add1/2
  L1/1 -> Product2/2
  lambda/1 -> Product/1
  L/1 -> Product1/1
  Product/1 -> Add/2
  wr/1 -> L1/1, L/1, Product/2
  1/L1/1 -> Integrator1/1
  Add1/1 -> 1/L1/1
  Integrator/1 -> r_wind/1, iq/1, Product2/1

== matlab function EV_compensated_system_via_detailed/Vehicle system/PMSM & Control Model/DQ Controller/MATLAB Function1 ==
  data: qd0 input; abc output; theta_r input
function abc = Inverse_DQTransform(qd0, theta_r)
%#codegen

Kr = 2/3*[  cos(theta_r)      cos(theta_r-2*pi/3)     cos(theta_r + 2*pi/3);
            sin(theta_r)      sin(theta_r-2*pi/3)     sin(theta_r + 2*pi/3);
            1/2               1/2                     1/2];
  
abc = Kr\qd0;

== matlab function EV_compensated_system_via_detailed/Vehicle system/PMSM & Control Model/DQ Controller/MATLAB Function ==
  data: abc input; qd0 output; theta_r input
function qd0 = DQTransform(abc, theta_r)
%#codegen

Kr = 2/3*[  cos(theta_r)      cos(theta_r-2*pi/3)     cos(theta_r + 2*pi/3);
            sin(theta_r)      sin(theta_r-2*pi/3)     sin(theta_r + 2*pi/3);
            1/2               1/2                     1/2];
  
qd0 = Kr*abc;

== matlab function EV_compensated_system_via_detailed/Vehicle system/PMSM & Control Model/PMSM/MATLAB Function ==
  data: abc input; qd0 output; theta_r input
function qd0 = DQTransform(abc, theta_r)
%#codegen

Kr = 2/3*[  cos(theta_r)      cos(theta_r-2*pi/3)     cos(theta_r + 2*pi/3);
            sin(theta_r)      sin(theta_r-2*pi/3)     sin(theta_r + 2*pi/3);
            1/2               1/2                     1/2];
  
qd0 = Kr*abc;

== matlab function EV_compensated_system_via_detailed/Vehicle system/PMSM & Control Model/PMSM/MATLAB Function1 ==
  data: qd0 input; abc output; theta_r input
function abc = Inverse_DQTransform(qd0, theta_r)
%#codegen

Kr = 2/3*[  cos(theta_r)      cos(theta_r-2*pi/3)     cos(theta_r + 2*pi/3);
            sin(theta_r)      sin(theta_r-2*pi/3)     sin(theta_r + 2*pi/3);
            1/2               1/2                     1/2];
  
abc = Kr\qd0;
